simulink model "MSRE_final_9region"  (R2017a)
settings: Solver=VariableStepAuto  StartTime=0.0  StopTime=5000  FixedStep=0.1  MaxStep=0.1
values from neighbouring files (symbols this model uses):
  a_f = -11.034E-5    (= -0.00011034)    [Parameters_U233_9region.m]    (also in Parameters_U235_9region.m = -8.71e-05)
  a_g = -05.814E-5    (= -5.814e-05)    [Parameters_U233_9region.m]    (also in Parameters_U235_9region.m = -6.66e-05)
  beta = [0.00023,0.00079,0.00067,0.00073,0.00013,0.00009]    [Parameters_U233_9region.m]    (also in Parameters_U235_9region.m = [0.000223,0.001457,0.001307,0.002628,0.000766,0.00023])
  beta_t = sum(beta)    [Parameters_U233_9region.m]    (also in Parameters_U235_9region.m)
  hA = [0.000392, 0.001204, 0.000900, 0.001174, 0.001977, 0.001525, 0.001985, 0.005445, 0.005360] * (9/5)    [Parameters_U233_9region.m]    (also in Parameters_U235_9region.m)
  hA_pn = ha_p/nn_s    (= 0.162)    [Parameters_U233_9region.m]    (also in Parameters_U235_9region.m)
  hA_rpn = h_roverall*A_rad/nn_rs    (= 0.000213033382331)    [Parameters_U233_9region.m]    (also in Parameters_U235_9region.m = 0.0170426705865)
  hA_rsn = h_roverall*A_rad/nn_rs    (= 0.000213033382331)    [Parameters_U233_9region.m]    (also in Parameters_U235_9region.m = 0.0170426705865)
  hA_sn = ha_s/nn_s    (= 0.0765)    [Parameters_U233_9region.m]    (also in Parameters_U235_9region.m)
  Ig = [0.04443, 0.08835, 0.16671, 0.12077, 0.09181, 0.17429, 0.12612, 0.08408, 0.10343]    [Parameters_U233_9region.m]    (also in Parameters_U235_9region.m)
  ka = [0.01493, 0.02736, 0.04504, 0.05126, 0.03601, 0.06014, 0.06845, 0.06179, 0.09333]    [Parameters_U233_9region.m]    (also in Parameters_U235_9region.m)
  kb = [0.01721, 0.04550, 0.04656, 0.04261, 0.06069, 0.06218, 0.05664, 0.07707, 0.07311]    [Parameters_U233_9region.m]    (also in Parameters_U235_9region.m)
  kga = [0.000946, 0.001685, 0.003029, 0.003447, 0.002216, 0.004044, 0.004603, 0.003920, 0.006277]    [Parameters_U233_9region.m]    (also in Parameters_U235_9region.m)
  kgb = [0.001081, 0.003060, 0.003131, 0.002395, 0.004081, 0.004182, 0.003184, 0.005183, 0.004305]    [Parameters_U233_9region.m]    (also in Parameters_U235_9region.m)
  Lam = 4.0E-04    (= 0.0004)    [Parameters_U233_9region.m]    (also in Parameters_U235_9region.m = 0.00024)
  lam = [1.260E-02, 3.370E-02, 1.390E-01, 3.250E-01, 1.130E+00, 2.500E+00]    [Parameters_U233_9region.m]    (also in Parameters_U235_9region.m = [1.240E-02, 3.05E-02, 1.11E-01, 3.01E-01, 1.140E+00, 3.014E+)
  m_fm = W_f * tau_m    (= 324.775986913)    [Parameters_U233_9region.m]    (also in Parameters_U235_9region.m)
  mcp_fa = [0.0151, 0.0512, 0.0280, 0.0350, 0.0866, 0.0473, 0.0592, 0.2380, 0.1615] * (9/5)    [Parameters_U233_9region.m]    (also in Parameters_U235_9region.m)
  mcp_fb = [0.0158, 0.0349, 0.0280, 0.0682, 0.0592, 0.0473, 0.1152, 0.1384, 0.2710] * (9/5)    [Parameters_U233_9region.m]    (also in Parameters_U235_9region.m)
  mcp_g = [0.0700, 0.2114, 0.1606, 0.2056, 0.3576, 0.2718, 0.3478, 0.9612, 0.9421] * (9/5)    [Parameters_U233_9region.m]    (also in Parameters_U235_9region.m)
  mcp_pn = mn_p*scp_p    (= 0.171276473487)    [Parameters_U233_9region.m]    (also in Parameters_U235_9region.m)
  mcp_rpn = mn_rp*cp_rp    (= 0.937931908109)    [Parameters_U233_9region.m]    (also in Parameters_U235_9region.m)
  mcp_rsn = mn_rs*scp_rs    (= 0.00358005261349)    [Parameters_U233_9region.m]    (also in Parameters_U235_9region.m)
  mcp_sn = mn_s*scp_s    (= 0.0595588455663)    [Parameters_U233_9region.m]    (also in Parameters_U235_9region.m)
  mcp_tn = m_tn*scp_t    (= 0.058453833323)    [Parameters_U233_9region.m]    (also in Parameters_U235_9region.m)
  mn_p = m_p/nn_p    (= 87.0971133928)    [Parameters_U233_9region.m]    (also in Parameters_U235_9region.m)
  mn_rp = m_rp/nn_rp    (= 392.440128916)    [Parameters_U233_9region.m]    (also in Parameters_U235_9region.m)
  mn_rs = m_rs/nn_rs    (= 3.549878645)    [Parameters_U233_9region.m]    (also in Parameters_U235_9region.m)
  mn_s = m_s/nn_s    (= 24.9200190654)    [Parameters_U233_9region.m]    (also in Parameters_U235_9region.m)
  n_frac0 = 1    [Parameters_U233_9region.m]    (also in Parameters_U235_9region.m)
  P = .1    (= 0.1)    [Parameters_U233_9region.m]    (also in Parameters_U235_9region.m = 8)
  T0_f1a = Tf_in + ((Ifa(1)/(Ifa(1)+Ifb(1)))*(Tf_out1-Tf_in))    [Parameters_U233_9region.m]    (also in Parameters_U235_9region.m)
  T0_f1b = T0_f1a + ((Ifb(1)/(Ifa(1)+Ifb(1)))*(Tf_out1-Tf_in))    [Parameters_U233_9region.m]    (also in Parameters_U235_9region.m)
  T0_f2a = Tf_in + ((Ifa(2)/(Ifa(2)+Ifb(2)+Ifa(3)+Ifb(3)+Ifa(4)+Ifb(4)))*(Tf_out2-Tf_in))    [Parameters_U233_9region.m]    (also in Parameters_U235_9region.m)
  T0_f2b = T0_f2a + ((Ifb(2)/(Ifa(2)+Ifb(2)+Ifa(3)+Ifb(3)+Ifa(4)+Ifb(4)))*(Tf_out2-Tf_in))    [Parameters_U233_9region.m]    (also in Parameters_U235_9region.m)
  T0_f3a = T0_f2b + ((Ifa(3)/(Ifa(2)+Ifb(2)+Ifa(3)+Ifb(3)+Ifa(4)+Ifb(4)))*(Tf_out2-Tf_in))    [Parameters_U233_9region.m]    (also in Parameters_U235_9region.m)
  T0_f3b = T0_f3a + ((Ifb(3)/(Ifa(2)+Ifb(2)+Ifa(3)+Ifb(3)+Ifa(4)+Ifb(4)))*(Tf_out2-Tf_in))    [Parameters_U233_9region.m]    (also in Parameters_U235_9region.m)
  T0_f4a = T0_f3b + ((Ifa(4)/(Ifa(2)+Ifb(2)+Ifa(3)+Ifb(3)+Ifa(4)+Ifb(4)))*(Tf_out2-Tf_in))    [Parameters_U233_9region.m]    (also in Parameters_U235_9region.m)
  T0_f4b = T0_f4a + ((Ifb(4)/(Ifa(2)+Ifb(2)+Ifa(3)+Ifb(3)+Ifa(4)+Ifb(4)))*(Tf_out2-Tf_in))    [Parameters_U233_9region.m]    (also in Parameters_U235_9region.m)
  T0_f5a = Tf_in + ((Ifa(5)/(Ifa(5)+Ifb(5)+Ifa(6)+Ifb(6)+Ifa(7)+Ifb(7)))*(Tf_out3-Tf_in))    [Parameters_U233_9region.m]    (also in Parameters_U235_9region.m)
  T0_f5b = T0_f5a + ((Ifb(5)/(Ifa(5)+Ifb(5)+Ifa(6)+Ifb(6)+Ifa(7)+Ifb(7)))*(Tf_out3-Tf_in))    [Parameters_U233_9region.m]    (also in Parameters_U235_9region.m)
  T0_f6a = T0_f5b + ((Ifa(6)/(Ifa(5)+Ifb(5)+Ifa(6)+Ifb(6)+Ifa(7)+Ifb(7)))*(Tf_out3-Tf_in))    [Parameters_U233_9region.m]    (also in Parameters_U235_9region.m)
  T0_f6b = T0_f6a + ((Ifb(6)/(Ifa(5)+Ifb(5)+Ifa(6)+Ifb(6)+Ifa(7)+Ifb(7)))*(Tf_out3-Tf_in))    [Parameters_U233_9region.m]    (also in Parameters_U235_9region.m)
  T0_f7a = T0_f6b + ((Ifa(7)/(Ifa(5)+Ifb(5)+Ifa(6)+Ifb(6)+Ifa(7)+Ifb(7)))*(Tf_out3-Tf_in))    [Parameters_U233_9region.m]    (also in Parameters_U235_9region.m)
  T0_f7b = T0_f7a + ((Ifb(7)/(Ifa(5)+Ifb(5)+Ifa(6)+Ifb(6)+Ifa(7)+Ifb(7)))*(Tf_out3-Tf_in))    [Parameters_U233_9region.m]    (also in Parameters_U235_9region.m)
  T0_f8a = Tf_in + ((Ifa(8)/(Ifa(8)+Ifb(8)+Ifa(9)+Ifb(9)))*(Tf_out4-Tf_in))    [Parameters_U233_9region.m]    (also in Parameters_U235_9region.m)
  T0_f8b = T0_f8a + ((Ifb(8)/(Ifa(8)+Ifb(8)+Ifa(9)+Ifb(9)))*(Tf_out4-Tf_in))    [Parameters_U233_9region.m]    (also in Parameters_U235_9region.m)
  T0_f9a = T0_f8b + ((Ifa(9)/(Ifa(8)+Ifb(8)+Ifa(9)+Ifb(9)))*(Tf_out4-Tf_in))    [Parameters_U233_9region.m]    (also in Parameters_U235_9region.m)
  T0_f9b = T0_f9a + ((Ifb(9)/(Ifa(8)+Ifb(8)+Ifa(9)+Ifb(9)))*(Tf_out4-Tf_in))    [Parameters_U233_9region.m]    (also in Parameters_U235_9region.m)
  T0_fm = Tf_out    (= 663.53)    [Parameters_U233_9region.m]    (also in Parameters_U235_9region.m)
  T0_g1 = T0_f1a+((kga(1)+kgb(1))*P/hA(1))    [Parameters_U233_9region.m]    (also in Parameters_U235_9region.m)
  T0_g2 = T0_f2a+((kga(2)+kgb(2))*P/hA(2))    [Parameters_U233_9region.m]    (also in Parameters_U235_9region.m)
  T0_g3 = T0_f3a+((kga(3)+kgb(3))*P/hA(3))    [Parameters_U233_9region.m]    (also in Parameters_U235_9region.m)
  T0_g4 = T0_f4a+((kga(4)+kgb(4))*P/hA(4))    [Parameters_U233_9region.m]    (also in Parameters_U235_9region.m)
  T0_g5 = T0_f5a+((kga(5)+kgb(5))*P/hA(5))    [Parameters_U233_9region.m]    (also in Parameters_U235_9region.m)
  T0_g6 = T0_f6a+((kga(6)+kgb(6))*P/hA(6))    [Parameters_U233_9region.m]    (also in Parameters_U235_9region.m)
  T0_g7 = T0_f7a+((kga(7)+kgb(7))*P/hA(7))    [Parameters_U233_9region.m]    (also in Parameters_U235_9region.m)
  T0_g8 = T0_f8a+((kga(8)+kgb(8))*P/hA(8))    [Parameters_U233_9region.m]    (also in Parameters_U235_9region.m)
  T0_g9 = T0_f9a+((kga(9)+kgb(9))*P/hA(9))    [Parameters_U233_9region.m]    (also in Parameters_U235_9region.m)
  T0_p1 = Tp_in - (Tp_in-T0_p2)/2    (= 647.875)    [Parameters_U233_9region.m]    (also in Parameters_U235_9region.m)
  T0_p2 = Tf_in    (= 632.22)    [Parameters_U233_9region.m]    (also in Parameters_U235_9region.m)
  T0_p3 = Tp_in - 3*(Tp_in-T0_p4)/4    (= 640.0475)    [Parameters_U233_9region.m]    (also in Parameters_U235_9region.m)
  T0_p4 = Tf_in    (= 632.22)    [Parameters_U233_9region.m]    (also in Parameters_U235_9region.m)
  T0_rp = Ts_in    (= 546.11)    [Parameters_U233_9region.m]    (also in Parameters_U235_9region.m)
  T0_rs = 148.9    [Parameters_U233_9region.m]    (also in Parameters_U235_9region.m)
  T0_s1 = Ts_in + (T0_s2 - Ts_in)/2    (= 562.75)    [Parameters_U233_9region.m]    (also in Parameters_U235_9region.m)
  T0_s2 = 5.7939E+02    (= 579.39)    [Parameters_U233_9region.m]    (also in Parameters_U235_9region.m)
  T0_s3 = Ts_in + 3*(T0_s4-Ts_in)/nn_s    (= 571.07)    [Parameters_U233_9region.m]    (also in Parameters_U235_9region.m)
  T0_s4 = 5.7939E+02    (= 579.39)    [Parameters_U233_9region.m]    (also in Parameters_U235_9region.m)
  T0_t1 = (T0_p1*hA_pn+T0_s3*hA_sn)/(hA_pn+hA_sn)    (= 628.556226415)    [Parameters_U233_9region.m]    (also in Parameters_U235_9region.m)
  T0_t2 = (T0_p3*hA_pn+T0_s1*hA_sn)/(hA_pn+hA_sn)    (= 612.585283019)    [Parameters_U233_9region.m]    (also in Parameters_U235_9region.m)
  tau_c = 8.46    [Parameters_U233_9region.m]    (also in Parameters_U235_9region.m)
  tau_c_hx = 3.77    [Parameters_U233_9region.m]    (also in Parameters_U235_9region.m)
  tau_fa = [1.386, 2.083, 1.139, 1.424, 2.084, 1.139, 1.424, 2.371, 1.610]    [Parameters_U233_9region.m]    (also in Parameters_U235_9region.m)
  tau_fb = [1.454, 1.424, 1.139, 2.772, 1.424, 1.139, 2.774, 1.380, 2.700]    [Parameters_U233_9region.m]    (also in Parameters_U235_9region.m)
  tau_hx_c = 8.67    [Parameters_U233_9region.m]    (also in Parameters_U235_9region.m)
  tau_hx_r = 4.71    [Parameters_U233_9region.m]    (also in Parameters_U235_9region.m)
  tau_l = 16.73    [Parameters_U233_9region.m]    (also in Parameters_U235_9region.m)
  tau_r_hx = 8.24    [Parameters_U233_9region.m]    (also in Parameters_U235_9region.m)
  Trs_in = 37.78    [Parameters_U233_9region.m]    (also in Parameters_U235_9region.m)
  W_f1 = (mcp_fa(1)/scp_f)/tau_fa(1)    [Parameters_U233_9region.m]    (also in Parameters_U235_9region.m)
  W_f2 = (mcp_fa(2)/scp_f)/tau_fa(2)    [Parameters_U233_9region.m]    (also in Parameters_U235_9region.m)
  W_f3 = (mcp_fa(5)/scp_f)/tau_fa(5)    [Parameters_U233_9region.m]    (also in Parameters_U235_9region.m)
  W_f4 = (mcp_fa(8)/scp_f)/tau_fa(8)    [Parameters_U233_9region.m]    (also in Parameters_U235_9region.m)
  W_p = W_f    (= 162.387993457)    [Parameters_U233_9region.m]    (also in Parameters_U235_9region.m)
  W_rp = W_s    (= 100.579336981)    [Parameters_U233_9region.m]    (also in Parameters_U235_9region.m)
  W_rs = 8.923430894987993e+01    (= 89.2343089499)    [Parameters_U233_9region.m]    (also in Parameters_U235_9region.m)
  W_s = 1.005793369810108e+02    (= 100.579336981)    [Parameters_U233_9region.m]    (also in Parameters_U235_9region.m)
undefined symbols (not defined in the file or in its folder): C0
settings Model: Creator=mlish  LastModifiedBy=VIKRAM SINGH

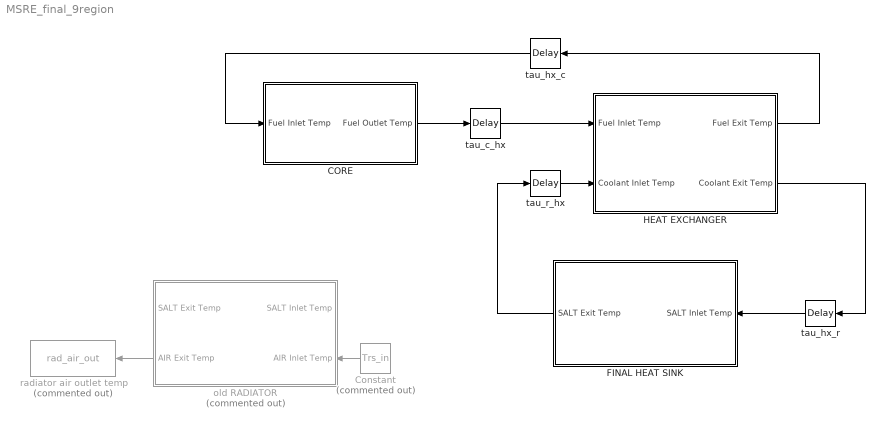
== system MSRE_final_9region ==
  " HEAT EXCHANGER" : Subsystem
  CORE : Subsystem
  Constant : Constant  Commented=on  Value=Trs_in
  FINAL HEAT SINK : Subsystem
  old RADIATOR : Subsystem  Commented=on
  radiator air outlet temp : ToWorkspace  Commented=on  VariableName=rad_air_out  SampleTime=-1
  tau_c_hx : TransportDelay  DelayTime=tau_c_hx  InitialOutput=T0_fm  BufferSize=4096
  tau_hx_c : TransportDelay  DelayTime=tau_hx_c  InitialOutput=T0_p4  BufferSize=4096
  tau_hx_r : TransportDelay  DelayTime=tau_hx_r  InitialOutput=T0_s4  BufferSize=4096
  tau_r_hx : TransportDelay  DelayTime=tau_r_hx  InitialOutput=T0_rp  BufferSize=4096
  wires:
  tau_c_hx/1 -> " HEAT EXCHANGER"/1(Fuel Inlet Temp)
  " HEAT EXCHANGER"/2(Coolant Exit Temp) -> tau_hx_r/1
  tau_hx_c/1 -> CORE/1(Fuel Inlet Temp)
  CORE/1(Fuel Outlet Temp) -> tau_c_hx/1
  tau_r_hx/1 -> " HEAT EXCHANGER"/2(Coolant Inlet Temp)
  " HEAT EXCHANGER"/1(Fuel Exit Temp) -> tau_hx_c/1
  old RADIATOR/2(AIR Exit Temp) -> radiator air outlet temp/1
  Constant/1 -> old RADIATOR/2(AIR Inlet Temp)
  tau_hx_r/1 -> FINAL HEAT SINK/1(SALT Inlet Temp)
  FINAL HEAT SINK/1(SALT Exit Temp) -> tau_r_hx/1

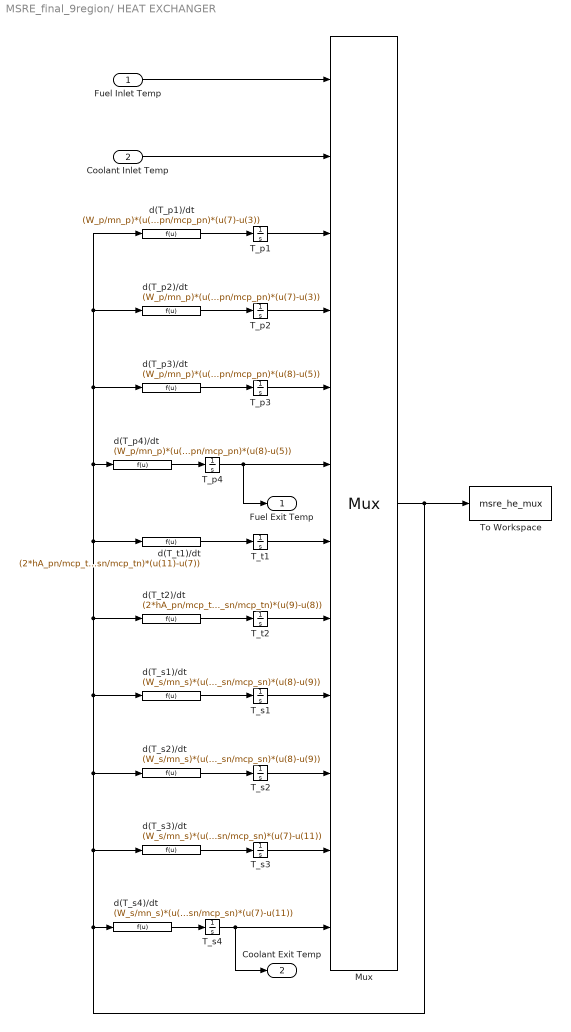
== system MSRE_final_9region/ HEAT EXCHANGER ==
  Fuel Inlet Temp : Inport
  Coolant Inlet Temp : Inport  Port=2
  Mux : Mux  Inputs=12
      settings: DisplayOption=signals
  T_p1 : Integrator  InitialCondition=T0_p1
  T_p2 : Integrator  InitialCondition=T0_p2
  "T_p3 " : Integrator  InitialCondition=T0_p3
  T_p4 : Integrator  InitialCondition=T0_p4
  T_s1 : Integrator  InitialCondition=T0_s1
  T_s2 : Integrator  InitialCondition=T0_s2
  T_s3 : Integrator  InitialCondition=T0_s3
  T_s4 : Integrator  InitialCondition=T0_s4
  T_t1 : Integrator  InitialCondition=T0_t1
  T_t2 : Integrator  InitialCondition=T0_t2
  To Workspace : ToWorkspace  VariableName=msre_he_mux  SampleTime=-1
  d(T_p1)/dt : Fcn  Expr=(W_p/mn_p)*(u(1)-u(3)) + (hA_pn/mcp_pn)*(u(7)-u(3))
  d(T_p2)/dt : Fcn  Expr=(W_p/mn_p)*(u(3)-u(4)) + (hA_pn/mcp_pn)*(u(7)-u(3))
  d(T_p3)/dt : Fcn  Expr=(W_p/mn_p)*(u(4)-u(5)) + (hA_pn/mcp_pn)*(u(8)-u(5))
  d(T_p4)/dt : Fcn  Expr=(W_p/mn_p)*(u(5)-u(6)) + (hA_pn/mcp_pn)*(u(8)-u(5))
  d(T_s1)/dt : Fcn  Expr=(W_s/mn_s)*(u(2)-u(9)) + (hA_sn/mcp_sn)*(u(8)-u(9))
  d(T_s2)/dt : Fcn  Expr=(W_s/mn_s)*(u(9)-u(10)) + (hA_sn/mcp_sn)*(u(8)-u(9))
  d(T_s3)/dt : Fcn  Expr=(W_s/mn_s)*(u(10)-u(11)) + (hA_sn/mcp_sn)*(u(7)-u(11))
  d(T_s4)/dt : Fcn  Expr=(W_s/mn_s)*(u(11)-u(12)) + (hA_sn/mcp_sn)*(u(7)-u(11))
  d(T_t1)/dt : Fcn  Expr=(2*hA_pn/mcp_tn)*(u(3)-u(7)) + (2*hA_sn/mcp_tn)*(u(11)-u(7))
  d(T_t2)/dt : Fcn  Expr=(2*hA_pn/mcp_tn)*(u(5)-u(8)) + (2*hA_sn/mcp_tn)*(u(9)-u(8))
  Fuel Exit Temp : Outport
  Coolant Exit Temp : Outport  Port=2
  wires:
  Fuel Inlet Temp/1 -> Mux/1
  Coolant Inlet Temp/1 -> Mux/2
  d(T_p1)/dt/1 -> T_p1/1
  d(T_p2)/dt/1 -> T_p2/1
  d(T_p3)/dt/1 -> "T_p3 "/1
  d(T_p4)/dt/1 -> T_p4/1
  d(T_t1)/dt/1 -> T_t1/1
  d(T_t2)/dt/1 -> T_t2/1
  d(T_s1)/dt/1 -> T_s1/1
  d(T_s2)/dt/1 -> T_s2/1
  T_p2/1 -> Mux/4
  T_p1/1 -> Mux/3
  d(T_s3)/dt/1 -> T_s3/1
  d(T_s4)/dt/1 -> T_s4/1
  Mux/1 -> d(T_s4)/dt/1, d(T_s3)/dt/1, d(T_s2)/dt/1, d(T_s1)/dt/1, d(T_t2)/dt/1, d(T_t1)/dt/1, d(T_p4)/dt/1, d(T_p3)/dt/1, d(T_p2)/dt/1, d(T_p1)/dt/1, To Workspace/1
  "T_p3 "/1 -> Mux/5
  T_p4/1 -> Fuel Exit Temp/1, Mux/6
  T_t1/1 -> Mux/7
  T_s4/1 -> Coolant Exit Temp/1, Mux/12
  T_s3/1 -> Mux/11
  T_s2/1 -> Mux/10
  T_s1/1 -> Mux/9
  T_t2/1 -> Mux/8

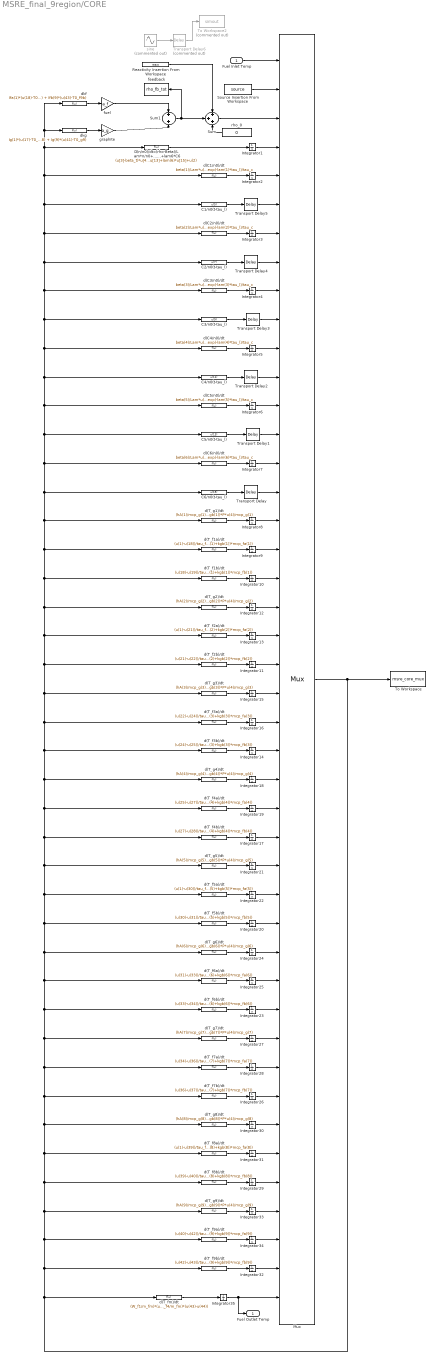
== system MSRE_final_9region/CORE ==
  Fuel Inlet Temp : Inport
  C1/n0(t-tau_l) : Fcn  Expr=u(5)
  C2/n0(t-tau_l) : Fcn  Expr=u(7)
  C3/n0(t-tau_l) : Fcn  Expr=u(9)
  C4/n0(t-tau_l) : Fcn  Expr=u(11)
  C5/n0(t-tau_l) : Fcn  Expr=u(13)
  C6/n0(t-tau_l) : Fcn  Expr=u(15)
  D(n/n0)/dt=(rho-Beta)/Lam*n/n0+lam1*C1+...+lam6*C6 : Fcn  Expr=(u[3]-beta_t)*u[4]/Lam+lam(1)*u[5]+lam(2)*u[7]+lam(3)*u[9]+lam(4)*u[11]+lam(5)*u[13]+lam(6)*u[15]+u(2)
  Integrator1 : Integrator  InitialCondition=n_frac0
  Integrator10 : Integrator  InitialCondition=T0_f1b
  Integrator11 : Integrator  InitialCondition=T0_f2b
  Integrator12 : Integrator  InitialCondition=T0_g2
  Integrator13 : Integrator  InitialCondition=T0_f2a
  Integrator14 : Integrator  InitialCondition=T0_f3b
  Integrator15 : Integrator  InitialCondition=T0_g3
  Integrator16 : Integrator  InitialCondition=T0_f3a
  Integrator17 : Integrator  InitialCondition=T0_f4b
  Integrator18 : Integrator  InitialCondition=T0_g4
  Integrator19 : Integrator  InitialCondition=T0_f4a
  Integrator2 : Integrator  InitialCondition=C0(1)
  Integrator20 : Integrator  InitialCondition=T0_f5b
  Integrator21 : Integrator  InitialCondition=T0_g5
  Integrator22 : Integrator  InitialCondition=T0_f5a
  Integrator23 : Integrator  InitialCondition=T0_f6b
  Integrator24 : Integrator  InitialCondition=T0_g6
  Integrator25 : Integrator  InitialCondition=T0_f6a
  Integrator26 : Integrator  InitialCondition=T0_f7b
  Integrator27 : Integrator  InitialCondition=T0_g7
  Integrator28 : Integrator  InitialCondition=T0_f7a
  Integrator29 : Integrator  InitialCondition=T0_f8b
  Integrator3 : Integrator  InitialCondition=C0(2)
  Integrator30 : Integrator  InitialCondition=T0_g8
  Integrator31 : Integrator  InitialCondition=T0_f8a
  Integrator32 : Integrator  InitialCondition=T0_f9b
  Integrator33 : Integrator  InitialCondition=T0_g9
  Integrator34 : Integrator  InitialCondition=T0_f9a
  Integrator35 : Integrator  InitialCondition=T0_fm
  Integrator4 : Integrator  InitialCondition=C0(3)
  Integrator5 : Integrator  InitialCondition=C0(4)
  Integrator6 : Integrator  InitialCondition=C0(5)
  Integrator7 : Integrator  InitialCondition=C0(6)
  Integrator8 : Integrator  InitialCondition=T0_g1
  Integrator9 : Integrator  InitialCondition=T0_f1a
  Mux : Mux  Inputs=44
      settings: DisplayOption=signals
  Reactivity Insertion From Workspace : FromWorkspace  VariableName=react  Interpolate=off  OutputAfterFinalValue=Holding final value
  Source Insertion From Workspace : FromWorkspace  VariableName=source  SampleTime=1  Interpolate=off  OutputAfterFinalValue=Holding final value
  Sum : Sum  Inputs=+++
  Sum1 : Sum
  To Workspace : ToWorkspace  VariableName=msre_core_mux  SampleTime=-1
  To Workspace2 : ToWorkspace  Commented=on  VariableName=simout  SampleTime=-1
  Transport Delay : TransportDelay  DelayTime=tau_l  InitialOutput=C0(6)  BufferSize=4096
  Transport Delay1 : TransportDelay  DelayTime=tau_l  InitialOutput=C0(5)  BufferSize=4096
  Transport Delay2 : TransportDelay  DelayTime=tau_l  InitialOutput=C0(4)  BufferSize=4096
  Transport Delay3 : TransportDelay  DelayTime=tau_l  InitialOutput=C0(3)  BufferSize=4096
  Transport Delay4 : TransportDelay  DelayTime=tau_l  InitialOutput=C0(2)  BufferSize=4096
  Transport Delay5 : TransportDelay  DelayTime=tau_l  InitialOutput=C0(1)  BufferSize=4096
  Transport Delay6 : TransportDelay  Commented=on  DelayTime=3000  BufferSize=4096
  d(C1/n0)/dt : Fcn  Expr=beta(1)/Lam*u(4)-lam(1)*u(5)-u(5)/tau_c+u(6)*exp(-lam(1)*tau_l)/tau_c
  d(C2/n0)/dt : Fcn  Expr=beta(2)/Lam*u(4)-lam(2)*u(7)-u(7)/tau_c+u(8)*exp(-lam(2)*tau_l)/tau_c
  d(C3/n0)/dt : Fcn  Expr=beta(3)/Lam*u(4)-lam(3)*u(9)-u(9)/tau_c+u(10)*exp(-lam(3)*tau_l)/tau_c
  d(C4/n0)/dt : Fcn  Expr=beta(4)/Lam*u(4)-lam(4)*u(11)-u(11)/tau_c+u(12)*exp(-lam(4)*tau_l)/tau_c
  d(C5/n0)/dt : Fcn  Expr=beta(5)/Lam*u(4)-lam(5)*u(13)-u(13)/tau_c+u(14)*exp(-lam(5)*tau_l)/tau_c
  d(C6/n0)/dt : Fcn  Expr=beta(6)/Lam*u(4)-lam(6)*u(15)-u(15)/tau_c+u(16)*exp(-lam(6)*tau_l)/tau_c
  d(T_f1a)/dt : Fcn  Expr=(u(1)-u(18))/tau_fa(1) + ka(1)*P*u(4)/mcp_fa(1) + kga(1)*hA(1)*(u(17)-u(18))/((kga(1)+kgb(1))*mcp_fa(1))
  d(T_f1b)/dt : Fcn  Expr=(u(18)-u(19))/tau_fb(1) + kb(1)*P*u(4)/mcp_fb(1) + kgb(1)*hA(1)*(u(17)-u(18))/((kga(1)+kgb(1))*mcp_fb(1))
  d(T_f2a)/dt : Fcn  Expr=(u(1)-u(21))/tau_fa(2) + ka(2)*P*u(4)/mcp_fa(2) + kga(2)*hA(2)*(u(20)-u(21))/((kga(2)+kgb(2))*mcp_fa(2))
  d(T_f2b)/dt : Fcn  Expr=(u(21)-u(22))/tau_fb(2) + kb(2)*P*u(4)/mcp_fb(2) + kgb(2)*hA(2)*(u(20)-u(21))/((kga(2)+kgb(2))*mcp_fb(2))
  d(T_f3a)/dt : Fcn  Expr=(u(22)-u(24))/tau_fa(3) + ka(3)*P*u(4)/mcp_fa(3) + kga(3)*hA(3)*(u(23)-u(24))/((kga(3)+kgb(3))*mcp_fa(3))
  d(T_f3b)/dt : Fcn  Expr=(u(24)-u(25))/tau_fb(3) + kb(3)*P*u(4)/mcp_fb(3) + kgb(3)*hA(3)*(u(23)-u(24))/((kga(3)+kgb(3))*mcp_fb(3))
  d(T_f4a)/dt : Fcn  Expr=(u(25)-u(27))/tau_fa(4) + ka(4)*P*u(4)/mcp_fa(4) + kga(4)*hA(4)*(u(26)-u(27))/((kga(4)+kgb(4))*mcp_fa(4))
  d(T_f4b)/dt : Fcn  Expr=(u(27)-u(28))/tau_fb(4) + kb(4)*P*u(4)/mcp_fb(4) + kgb(4)*hA(4)*(u(26)-u(27))/((kga(4)+kgb(4))*mcp_fb(4))
  d(T_f5a)/dt : Fcn  Expr=(u(1)-u(30))/tau_fa(5) + ka(5)*P*u(4)/mcp_fa(5) + kga(5)*hA(5)*(u(29)-u(30))/((kga(5)+kgb(5))*mcp_fa(5))
  d(T_f5b)/dt : Fcn  Expr=(u(30)-u(31))/tau_fb(5) + kb(5)*P*u(4)/mcp_fb(5) + kgb(5)*hA(5)*(u(29)-u(30))/((kga(5)+kgb(5))*mcp_fb(5))
  d(T_f6a)/dt : Fcn  Expr=(u(31)-u(33))/tau_fa(6) + ka(6)*P*u(4)/mcp_fa(6) + kga(6)*hA(6)*(u(32)-u(33))/((kga(6)+kgb(6))*mcp_fa(6))
  d(T_f6b)/dt : Fcn  Expr=(u(33)-u(34))/tau_fb(6) + kb(6)*P*u(4)/mcp_fb(6) + kgb(6)*hA(6)*(u(32)-u(33))/((kga(6)+kgb(6))*mcp_fb(6))
  d(T_f7a)/dt : Fcn  Expr=(u(34)-u(36))/tau_fa(7) + ka(7)*P*u(4)/mcp_fa(7) + kga(7)*hA(7)*(u(35)-u(36))/((kga(7)+kgb(7))*mcp_fa(7))
  d(T_f7b)/dt : Fcn  Expr=(u(36)-u(37))/tau_fb(7) + kb(7)*P*u(4)/mcp_fb(7) + kgb(7)*hA(7)*(u(35)-u(36))/((kga(7)+kgb(7))*mcp_fb(7))
  d(T_f8a)/dt : Fcn  Expr=(u(1)-u(39))/tau_fa(8) + ka(8)*P*u(4)/mcp_fa(8) + kga(8)*hA(8)*(u(38)-u(39))/((kga(8)+kgb(8))*mcp_fa(8))
  d(T_f8b)/dt : Fcn  Expr=(u(39)-u(40))/tau_fb(8) + kb(8)*P*u(4)/mcp_fb(8) + kgb(8)*hA(8)*(u(38)-u(39))/((kga(8)+kgb(8))*mcp_fb(8))
  d(T_f9a)/dt : Fcn  Expr=(u(40)-u(42))/tau_fa(9) + ka(9)*P*u(4)/mcp_fa(9) + kga(9)*hA(9)*(u(41)-u(42))/((kga(9)+kgb(9))*mcp_fa(9))
  d(T_f9b)/dt : Fcn  Expr=(u(42)-u(43))/tau_fb(9) + kb(9)*P*u(4)/mcp_fb(9) + kgb(9)*hA(9)*(u(41)-u(42))/((kga(9)+kgb(9))*mcp_fb(9))
  d(T_fm)/dt : Fcn  Expr=(W_f1/m_fm)*(u(19)-u(44)) + (W_f2/m_fm)*(u(28)-u(44)) + (W_f3/m_fm)*(u(37)-u(44)) + (W_f4/m_fm)*(u(43)-u(44))
  d(T_g1)/dt : Fcn  Expr=(hA(1)/mcp_g(1))*(u(18)-u(17)) + (kga(1)+kgb(1))*P*u(4)/mcp_g(1)
  d(T_g2)/dt : Fcn  Expr=(hA(2)/mcp_g(2))*(u(21)-u(20)) + (kga(2)+kgb(2))*P*u(4)/mcp_g(2)
  d(T_g3)/dt : Fcn  Expr=(hA(3)/mcp_g(3))*(u(24)-u(23)) + (kga(3)+kgb(3))*P*u(4)/mcp_g(3)
  d(T_g4)/dt : Fcn  Expr=(hA(4)/mcp_g(4))*(u(27)-u(26)) + (kga(4)+kgb(4))*P*u(4)/mcp_g(4)
  d(T_g5)/dt : Fcn  Expr=(hA(5)/mcp_g(5))*(u(30)-u(29)) + (kga(5)+kgb(5))*P*u(4)/mcp_g(5)
  d(T_g6)/dt : Fcn  Expr=(hA(6)/mcp_g(6))*(u(33)-u(32)) + (kga(6)+kgb(6))*P*u(4)/mcp_g(6)
  d(T_g7)/dt : Fcn  Expr=(hA(7)/mcp_g(7))*(u(36)-u(35)) + (kga(7)+kgb(7))*P*u(4)/mcp_g(7)
  d(T_g8)/dt : Fcn  Expr=(hA(8)/mcp_g(8))*(u(39)-u(38)) + (kga(8)+kgb(8))*P*u(4)/mcp_g(8)
  d(T_g9)/dt : Fcn  Expr=(hA(9)/mcp_g(9))*(u(42)-u(41)) + (kga(9)+kgb(9))*P*u(4)/mcp_g(9)
  dkf : Fcn  Expr=Ifa(1)*(u(18)-T0_f1a) + Ifb(1)*(u(19)-T0_f1b) + Ifa(2)*(u(21)-T0_f2a) + Ifb(2)*(u(22)-T0_f2b) + Ifa(3)*(u(24)-T0_f3a) + Ifb(3)*(u(25)-T0_f3b) + Ifa(4)*(u(27)-T0_f4a) + Ifb(4)*(u(28)-T0_f4b) + Ifa(5)*(u(30)-T0_f5a) + Ifb(5)*(u(31)-T0_f5b) + Ifa(6)*(u(33)-T0_f6a) + Ifb(6)*(u(34)-T0_f6b) + Ifa(7)*(u(36)-T0_f7a) + Ifb(7)*(u(37)-T0_f7b) + Ifa(8)*(u(39)-T0_f8a) + Ifb(8)*(u(40)-T0_f8b) + Ifa(9)*(u(42)-T0_f9a) + Ifb(9)*(u(43)-T0_f9b)
  dkg : Fcn  Expr=Ig(1)*(u(17)-T0_g1) + Ig(2)*(u(20)-T0_g2) + Ig(3)*(u(23)-T0_g3) + Ig(4)*(u(26)-T0_g4) + Ig(5)*(u(29)-T0_g5) + Ig(6)*(u(32)-T0_g6) + Ig(7)*(u(35)-T0_g7) + Ig(8)*(u(38)-T0_g8) + Ig(9)*(u(41)-T0_g9)
  feedback : ToWorkspace  VariableName=rho_fb_tot  SampleTime=-1
  fuel : Gain  Gain=a_f
  graphite : Gain  Gain=a_g
  rho_0 : Constant  Value=0
  sine : Sin  Commented=on  Amplitude=.1e-4  SampleTime=0
  Fuel Outlet Temp : Outport
  wires:
  Transport Delay3/1 -> Mux/10
  C3/n0(t-tau_l)/1 -> Transport Delay3/1
  Transport Delay4/1 -> Mux/8
  C4/n0(t-tau_l)/1 -> Transport Delay2/1
  Integrator7/1 -> Mux/15
  Transport Delay2/1 -> Mux/12
  C5/n0(t-tau_l)/1 -> Transport Delay1/1
  Transport Delay/1 -> Mux/16
  Transport Delay1/1 -> Mux/14
  C6/n0(t-tau_l)/1 -> Transport Delay/1
  D(n/n0)/dt=(rho-Beta)/Lam*n/n0+lam1*C1+...+lam6*C6/1 -> Integrator1/1
  d(C5/n0)/dt/1 -> Integrator6/1
  d(C3/n0)/dt/1 -> Integrator4/1
  d(C2/n0)/dt/1 -> Integrator3/1
  d(C4/n0)/dt/1 -> Integrator5/1
  d(C1/n0)/dt/1 -> Integrator2/1
  C2/n0(t-tau_l)/1 -> Transport Delay4/1
  Source Insertion From Workspace/1 -> Mux/2
  C1/n0(t-tau_l)/1 -> Transport Delay5/1
  Transport Delay5/1 -> Mux/6
  d(C6/n0)/dt/1 -> Integrator7/1
  Integrator5/1 -> Mux/11
  Integrator3/1 -> Mux/7
  Integrator2/1 -> Mux/5
  Integrator4/1 -> Mux/9
  Integrator1/1 -> Mux/4
  Integrator6/1 -> Mux/13
  d(T_f1b)/dt/1 -> Integrator10/1
  d(T_f1a)/dt/1 -> Integrator9/1
  d(T_g1)/dt/1 -> Integrator8/1
  Fuel Inlet Temp/1 -> Mux/1
  d(T_f2a)/dt/1 -> Integrator13/1
  d(T_f2b)/dt/1 -> Integrator11/1
  d(T_g2)/dt/1 -> Integrator12/1
  d(T_g3)/dt/1 -> Integrator15/1
  d(T_f3b)/dt/1 -> Integrator14/1
  d(T_f3a)/dt/1 -> Integrator16/1
  d(T_f4a)/dt/1 -> Integrator19/1
  d(T_g4)/dt/1 -> Integrator18/1
  d(T_f4b)/dt/1 -> Integrator17/1
  d(T_f5a)/dt/1 -> Integrator22/1
  d(T_g5)/dt/1 -> Integrator21/1
  d(T_f5b)/dt/1 -> Integrator20/1
  d(T_f6a)/dt/1 -> Integrator25/1
  d(T_g6)/dt/1 -> Integrator24/1
  d(T_f6b)/dt/1 -> Integrator23/1
  d(T_f7a)/dt/1 -> Integrator28/1
  d(T_g7)/dt/1 -> Integrator27/1
  d(T_f7b)/dt/1 -> Integrator26/1
  d(T_f8a)/dt/1 -> Integrator31/1
  d(T_g8)/dt/1 -> Integrator30/1
  d(T_f8b)/dt/1 -> Integrator29/1
  d(T_f9a)/dt/1 -> Integrator34/1
  d(T_g9)/dt/1 -> Integrator33/1
  d(T_f9b)/dt/1 -> Integrator32/1
  d(T_fm)/dt/1 -> Integrator35/1
  Mux/1 -> To Workspace/1, d(T_fm)/dt/1, d(T_f9b)/dt/1, d(T_f9a)/dt/1, d(T_g9)/dt/1, d(T_f8b)/dt/1, d(T_f8a)/dt/1, d(T_g8)/dt/1, d(T_f7b)/dt/1, d(T_f7a)/dt/1, d(T_g7)/dt/1, d(T_f6b)/dt/1, d(T_f6a)/dt/1, d(T_g6)/dt/1, d(T_f5b)/dt/1, d(T_f5a)/dt/1, d(T_g5)/dt/1, d(T_f4b)/dt/1, d(T_f4a)/dt/1, d(T_g4)/dt/1, d(T_f3b)/dt/1, d(T_f3a)/dt/1, d(T_g3)/dt/1, d(T_f2b)/dt/1, d(T_f2a)/dt/1, d(T_g2)/dt/1, d(T_f1b)/dt/1, d(T_f1a)/dt/1, C6/n0(t-tau_l)/1, d(C6/n0)/dt/1, C5/n0(t-tau_l)/1, d(C5/n0)/dt/1, C4/n0(t-tau_l)/1, d(C4/n0)/dt/1, C3/n0(t-tau_l)/1, d(C3/n0)/dt/1, d(C2/n0)/dt/1, dkf/1, dkg/1, D(n/n0)/dt=(rho-Beta)/Lam*n/n0+lam1*C1+...+lam6*C6/1, d(C1/n0)/dt/1, C1/n0(t-tau_l)/1, C2/n0(t-tau_l)/1, d(T_g1)/dt/1
  Integrator8/1 -> Mux/17
  Integrator9/1 -> Mux/18
  Integrator10/1 -> Mux/19
  Integrator12/1 -> Mux/20
  Integrator13/1 -> Mux/21
  Integrator11/1 -> Mux/22
  Integrator15/1 -> Mux/23
  Integrator16/1 -> Mux/24
  Integrator14/1 -> Mux/25
  Integrator18/1 -> Mux/26
  Integrator19/1 -> Mux/27
  Integrator17/1 -> Mux/28
  Integrator21/1 -> Mux/29
  Integrator22/1 -> Mux/30
  Integrator20/1 -> Mux/31
  Integrator24/1 -> Mux/32
  Integrator25/1 -> Mux/33
  Integrator23/1 -> Mux/34
  Integrator27/1 -> Mux/35
  Integrator28/1 -> Mux/36
  Integrator26/1 -> Mux/37
  Integrator30/1 -> Mux/38
  Integrator31/1 -> Mux/39
  Integrator29/1 -> Mux/40
  Integrator33/1 -> Mux/41
  Integrator34/1 -> Mux/42
  Integrator32/1 -> Mux/43
  Integrator35/1 -> Fuel Outlet Temp/1, Mux/44
  dkf/1 -> fuel/1
  dkg/1 -> graphite/1
  Sum/1 -> Mux/3
  Transport Delay6/1 -> To Workspace2/1
  sine/1 -> Transport Delay6/1
  fuel/1 -> Sum1/1
  graphite/1 -> Sum1/2
  Sum1/1 -> Sum/2, feedback/1
  rho_0/1 -> Sum/3
  Reactivity Insertion From Workspace/1 -> Sum/1

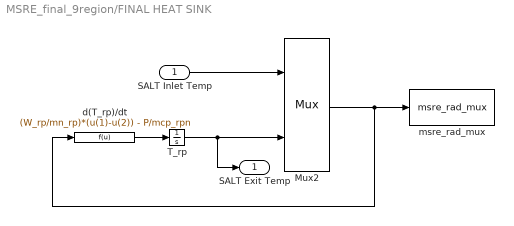
== system MSRE_final_9region/FINAL HEAT SINK ==
  SALT Inlet Temp : Inport
  Mux2 : Mux  Inputs=2
      settings: DisplayOption=signals
  T_rp : Integrator  InitialCondition=T0_rp
  d(T_rp)/dt : Fcn  Expr=(W_rp/mn_rp)*(u(1)-u(2)) - P/mcp_rpn
  msre_rad_mux : ToWorkspace  VariableName=msre_rad_mux  SampleTime=-1
  SALT Exit Temp : Outport
  wires:
  SALT Inlet Temp/1 -> Mux2/1
  d(T_rp)/dt/1 -> T_rp/1
  T_rp/1 -> SALT Exit Temp/1, Mux2/2
  Mux2/1 -> d(T_rp)/dt/1, msre_rad_mux/1

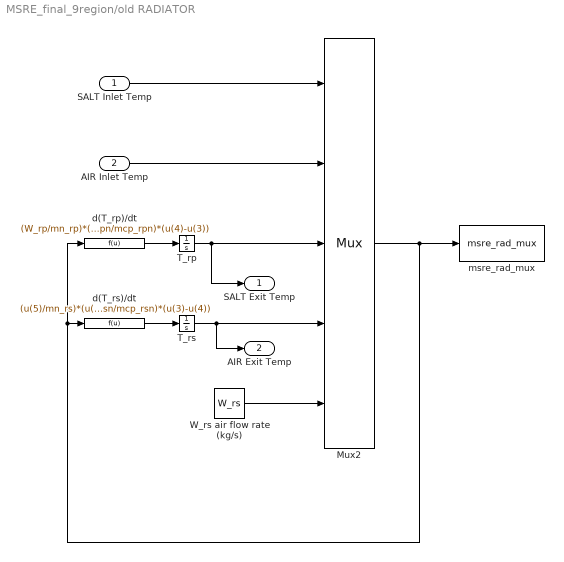
== system MSRE_final_9region/old RADIATOR ==
  SALT Inlet Temp : Inport
  AIR Inlet Temp : Inport  Port=2
  Mux2 : Mux  Inputs=5
      settings: DisplayOption=signals
  T_rp : Integrator  InitialCondition=T0_rp
  T_rs : Integrator  InitialCondition=T0_rs
  W_rs air flow rate (kg/s) : Constant  Value=W_rs
  d(T_rp)/dt : Fcn  Expr=(W_rp/mn_rp)*(u(1)-u(3)) + (hA_rpn/mcp_rpn)*(u(4)-u(3))
  d(T_rs)/dt : Fcn  Expr=(u(5)/mn_rs)*(u(2)-u(4)) + (hA_rsn/mcp_rsn)*(u(3)-u(4))
  msre_rad_mux : ToWorkspace  VariableName=msre_rad_mux  SampleTime=-1
  SALT Exit Temp : Outport
  AIR Exit Temp : Outport  Port=2
  wires:
  SALT Inlet Temp/1 -> Mux2/1
  AIR Inlet Temp/1 -> Mux2/2
  d(T_rp)/dt/1 -> T_rp/1
  T_rp/1 -> Mux2/3, SALT Exit Temp/1
  d(T_rs)/dt/1 -> T_rs/1
  T_rs/1 -> Mux2/4, AIR Exit Temp/1
  Mux2/1 -> d(T_rs)/dt/1, d(T_rp)/dt/1, msre_rad_mux/1
  W_rs air flow rate (kg/s)/1 -> Mux2/5
